simulink model "PSPWM"  (R2013a)
settings: Solver=ode45  StartTime=0.0  StopTime=10.0  RelTol=1e-3
libraries: simulink x8, powerlib_meascontrol x6
settings Model: Creator=ASUS  LastModifiedBy=ASUS

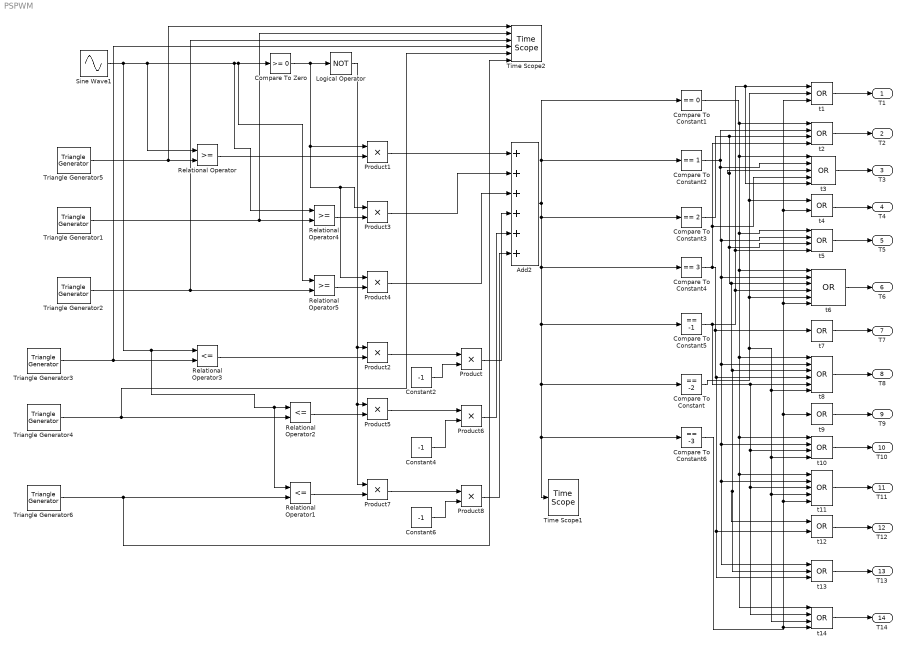
== system PSPWM ==
  Add2 : Sum  Inputs=++++++
  Compare To Constant : simulink/Logic and Bit Operations/Compare To Constant  relop===  const=-2  OutDataTypeStr=boolean
  Compare To Constant1 : simulink/Logic and Bit Operations/Compare To Constant  relop===  const=0  OutDataTypeStr=boolean
  Compare To Constant2 : simulink/Logic and Bit Operations/Compare To Constant  relop===  const=1  OutDataTypeStr=boolean
  Compare To Constant3 : simulink/Logic and Bit Operations/Compare To Constant  relop===  const=2  OutDataTypeStr=boolean
  Compare To Constant4 : simulink/Logic and Bit Operations/Compare To Constant  relop===  const=3  OutDataTypeStr=boolean
  Compare To Constant5 : simulink/Logic and Bit Operations/Compare To Constant  relop===  const=-1  OutDataTypeStr=boolean
  Compare To Constant6 : simulink/Logic and Bit Operations/Compare To Constant  relop===  const=-3  OutDataTypeStr=boolean
  Compare To Zero : simulink/Logic and Bit Operations/Compare To Zero  relop=>=  OutDataTypeStr=boolean
  Constant2 : Constant  Value=-1
  Constant4 : Constant  Value=-1
  Constant6 : Constant  Value=-1
  Logical Operator : Logic  Operator=NOT  AllPortsSameDT=off  OutDataTypeStr=boolean
  Product{,1..8} (9 alike) : Product
  Relational Operator : RelationalOperator  OutDataTypeStr=boolean  ZeroCross=off
  Relational Operator1 : RelationalOperator  Operator=<=  OutDataTypeStr=boolean
  Relational Operator2 : RelationalOperator  Operator=<=  OutDataTypeStr=boolean
  Relational Operator3 : RelationalOperator  Operator=<=  OutDataTypeStr=boolean
  Relational Operator4 : RelationalOperator  OutDataTypeStr=boolean  ZeroCross=off
  Relational Operator5 : RelationalOperator  OutDataTypeStr=boolean  ZeroCross=off
  Sine Wave1 : Sin  Amplitude=3  Frequency=2*pi*50  SampleTime=0
  Time Scope1 : TimeScope  DefaultConfigurationName=spbscopes.TimeScopeBlockCfg
      settings: CopyFcn=scopeextensions.ScopeBlock.callback(gcbh, 'onBlockCopy', gcbh);  DeleteFcn=scopeextensions.ScopeBlock.callback(gcbh, 'onBlockDelete');  PreSaveFcn=scopeextensions.ScopeBlock.callback(gcbh, 'onModelSave');  NameChangeFcn=scopeextensions.ScopeBlock.callback(gcbh, 'onBlockRename');  CloseFcn=scopeextensions.ScopeBlock.callback(gcbh, 'onBlockClose');  PreDeleteFcn=scopeextensions.ScopeBlock.callback(gcbh, 'onBlockPreDelete');
  Time Scope2 : TimeScope  NumInputPorts=6  DefaultConfigurationName=spbscopes.TimeScopeBlockCfg
      settings: CopyFcn=scopeextensions.ScopeBlock.callback(gcbh, 'onBlockCopy', gcbh);  DeleteFcn=scopeextensions.ScopeBlock.callback(gcbh, 'onBlockDelete');  PreSaveFcn=scopeextensions.ScopeBlock.callback(gcbh, 'onModelSave');  NameChangeFcn=scopeextensions.ScopeBlock.callback(gcbh, 'onBlockRename');  CloseFcn=scopeextensions.ScopeBlock.callback(gcbh, 'onBlockClose');  PreDeleteFcn=scopeextensions.ScopeBlock.callback(gcbh, 'onBlockPreDelete');
  Triangle Generator1 : powerlib_meascontrol/Pulse & Signal Generators/Triangle Generator  Freq=800  Phase=60  Ts=0
      link override Model/Continuous/Constant2: Value=0
      link override Model/Continuous/Lookup Table: Table=[-3 3 -3]
  Triangle Generator2 : powerlib_meascontrol/Pulse & Signal Generators/Triangle Generator  Freq=800  Phase=120  Ts=0
      link override Model/Continuous/Constant2: Value=0
      link override Model/Continuous/Lookup Table: Table=[-3 3 -3]
  Triangle Generator3 : powerlib_meascontrol/Pulse & Signal Generators/Triangle Generator  Freq=800  Phase=0  Ts=0
      link override Model/Continuous/Constant2: Value=0
      link override Model/Continuous/Lookup Table: Table=[3 -3 3]
  Triangle Generator4 : powerlib_meascontrol/Pulse & Signal Generators/Triangle Generator  Freq=800  Phase=60  Ts=0
      link override Model/Continuous/Constant2: Value=0
      link override Model/Continuous/Lookup Table: Table=[3 -3 3]
  Triangle Generator5 : powerlib_meascontrol/Pulse & Signal Generators/Triangle Generator  Freq=800  Phase=0  Ts=0
      link override Model/Continuous/Constant2: Value=0
      link override Model/Continuous/Lookup Table: Table=[-3 3 -3]
  Triangle Generator6 : powerlib_meascontrol/Pulse & Signal Generators/Triangle Generator  Freq=800  Phase=120  Ts=0
      link override Model/Continuous/Constant2: Value=0
      link override Model/Continuous/Lookup Table: Table=[3 -3 3]
  t1 : Logic  Operator=OR  Inputs=3  AllPortsSameDT=off  OutDataTypeStr=boolean
  t{2,5,10,14} (4 alike) : Logic  Operator=OR  Inputs=4  AllPortsSameDT=off  OutDataTypeStr=boolean
  t11 : Logic  Operator=OR  Inputs=5  AllPortsSameDT=off  OutDataTypeStr=boolean
  t12 : Logic  Operator=OR  AllPortsSameDT=off  OutDataTypeStr=boolean
  t13 : Logic  Operator=OR  Inputs=3  AllPortsSameDT=off  OutDataTypeStr=boolean
  t3 : Logic  Operator=OR  Inputs=5  AllPortsSameDT=off  OutDataTypeStr=boolean
  t4 : Logic  Operator=OR  AllPortsSameDT=off  OutDataTypeStr=boolean
  t6 : Logic  Operator=OR  Inputs=6  AllPortsSameDT=off  OutDataTypeStr=boolean
  t7 : Logic  Operator=OR  Inputs=1  AllPortsSameDT=off  OutDataTypeStr=boolean
  t8 : Logic  Operator=OR  Inputs=6  AllPortsSameDT=off  OutDataTypeStr=boolean
  t9 : Logic  Operator=OR  Inputs=1  AllPortsSameDT=off  OutDataTypeStr=boolean
  T1 : Outport
  T2 : Outport  Port=2
  T3 : Outport  Port=3
  T4 : Outport  Port=4
  T5 : Outport  Port=5
  T6 : Outport  Port=6
  T7 : Outport  Port=7
  T8 : Outport  Port=8
  T9 : Outport  Port=9
  T10 : Outport  Port=10
  T11 : Outport  Port=11
  T12 : Outport  Port=12
  T13 : Outport  Port=13
  T14 : Outport  Port=14
  wires:
  Sine Wave1/1 -> Relational Operator1/1, Relational Operator2/1, Relational Operator3/1, Relational Operator/1, Relational Operator4/1, Relational Operator5/1, Compare To Zero/1
  Compare To Zero/1 -> Product4/1, Product3/1, Product1/1, Logical Operator/1
  Relational Operator/1 -> Product1/2
  Triangle Generator1/1 -> Time Scope2/2, Relational Operator4/2
  Relational Operator4/1 -> Product3/2
  Triangle Generator2/1 -> Time Scope2/3, Relational Operator5/2
  Relational Operator5/1 -> Product4/2
  Product1/1 -> Add2/1
  Product3/1 -> Add2/2
  Triangle Generator3/1 -> Time Scope2/4, Relational Operator3/2
  Relational Operator3/1 -> Product2/2
  Logical Operator/1 -> Product7/1, Product5/1, Product2/1
  Constant2/1 -> Product/2
  Product2/1 -> Product/1
  Triangle Generator4/1 -> Time Scope2/5, Relational Operator2/2
  Relational Operator2/1 -> Product5/2
  Constant4/1 -> Product6/2
  Product5/1 -> Product6/1
  Triangle Generator6/1 -> Time Scope2/6, Relational Operator1/2
  Relational Operator1/1 -> Product7/2
  Product7/1 -> Product8/1
  Constant6/1 -> Product8/2
  Add2/1 -> Compare To Constant2/1, Compare To Constant1/1, Compare To Constant3/1, Compare To Constant4/1, Compare To Constant5/1, Compare To Constant6/1, Time Scope1/1, Compare To Constant/1
  Triangle Generator5/1 -> Time Scope2/1, Relational Operator/2
  Product4/1 -> Add2/3
  Product/1 -> Add2/4
  Product6/1 -> Add2/5
  Product8/1 -> Add2/6
  Compare To Constant1/1 -> t5/1, t6/1, t8/1, t10/1, t11/1, t14/1, t3/1, t2/1
  Compare To Constant2/1 -> t2/2, t8/2, t11/2, t13/1, t10/2, t6/2, t5/2, t3/2
  Compare To Constant3/1 -> t13/2, t12/1, t8/3, t6/3, t5/3, t3/3, t2/3
  Compare To Constant4/1 -> t13/3, t12/2, t8/4, t7/1, t3/4, t2/4
  Compare To Constant5/1 -> t14/2, t11/3, t10/3, t8/5, t6/4, t5/4, t3/5, t1/1
  Compare To Constant/1 -> t14/3, t11/4, t10/4, t8/6, t6/5, t1/2, t4/1
  Compare To Constant6/1 -> t14/4, t11/5, t9/1, t6/6, t4/2, t1/3
  t1/1 -> T1/1
  t2/1 -> T2/1
  t3/1 -> T3/1
  t4/1 -> T4/1
  t5/1 -> T5/1
  t6/1 -> T6/1
  t7/1 -> T7/1
  t8/1 -> T8/1
  t9/1 -> T9/1
  t10/1 -> T10/1
  t11/1 -> T11/1
  t12/1 -> T12/1
  t13/1 -> T13/1
  t14/1 -> T14/1
